simulink library "xrbsImage_r3"  (Simulink 5.1)
libraries: xbsIndex_r3 x24, xrbsDSP_r3 x5, xrbsImage_r3 x4
settings Model: Creator=singhj  LastModifiedBy=shirazi  ProdHWDeviceType=Microprocessor

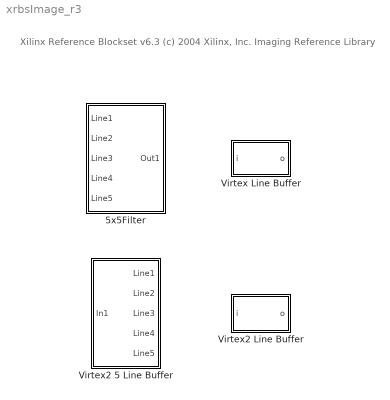
== system xrbsImage_r3 ==
  note: Xilinx Reference Blockset v6.3
      | (c) 2004  Xilinx, Inc.
      |
      | Imaging Reference Library
  5x5Filter : Subsystem  mask(5x5 Filter){maskNum=Edge, coef_n_bits=6, coef_bin_pt=0, smpl_n_bits=8, smpl_bin_pt=0, smpl_period=1, mask=0, maskDiv=0}
      mask prompts: maskNum "5x5 Mask"; coef_n_bits "Number of Bits per Coefficient"; coef_bin_pt "Binary Point for Coefficient"; smpl_n_bits "Number of Bits per Input Sample"; smpl_bin_pt "Binary Point for Input Samples"; smpl_period "Sample Period"; mask "Mask Value"; maskDiv "Mask Division"
      mask help: The Xilinx 5x5 Filter reference block is implemented using 5 n-tap MAC FIR Filters. Nine different 2-D filters have been provided to filter grayscale images.
      mask init:
      | [bg,fg] = xlcmap('XBlock',0);
      | iPos = get_param(gcb,'Position');
      | iWidth=iPos(3)-iPos(1); iHeight=iPos(4)-iPos(2);
      | iCx=iWidth/2;
      | iCy=iHeight/2;
      | [logoX, logoY] = xlogo(iPos);
      | 
      | % Different 5x5 Filters 
      | %  by default edge is used
      | 
      | edge = [ 0  0  0  0 0; ...
      |          0 -1 -1 -1 0; ...
      |          0 -1  8 -1 0; ...
      |          0 -1 -1 -1 0; ...
      |          0  0  0  0 0];
      | edgeDiv = 1;
      | 
      | sobelX = [ 0  0  0  0 0; ...
      |            0 -1  0  1 0; ...
      |            0 -2  0  2 0; ...
      |            0 -1  0  1 0; ...
      |            0  0  0  0 0];
      | sobelXDiv = 1;
      | 
      | sobelY = [ 0  0  0  0 0; ...
      |            0  1  2  1 0; ...
      |            0  0  0  0 0; ...
      |            0 -1 -2 -1 0; ...
      |            0  0  0  0 0];
      | sobelYDiv = 1;
      | 
      | sobelXY = [ 0  0  0  0 0; ...
      |             0  0 -1 -1 0; ...
      |             0  1  0 -1 0; ...
      |             0  1  1  0 0; ...
      |             0  0  0  0 0];
      | sobelXYDiv = 1;
      | 
      | blur = [ 1  1  1  1 1; ...
      |          1  0  0  0 1; ...
      |          1  0  0  0 1; ...
      |          1  0  0  0 1; ...
      |          1  1  1  1 1];
      | blurDiv = 1/16;
      | 
      | smooth = [ 1  1  1  1 1; ...
      |            1  5  5  5 1; ...
      |            1  5 44  5 1; ...
      |            1  5  5  5 1; ...
      |            1  1  1  1 1];
      | smoothDiv = 1/100;
      | 
      | sharpen = [ 0  0  0  0 0; ...
      |             0 -2 -2 -2 0; ...
      |             0 -2 32 -2 0; ...
      |             0 -2 -2 -2 0; ...
      |             0  0  0  0 0];
      | sharpenDiv = 1/16;
      | 
      | 
      | gaussian = [1 1 2 1 1; ...
      |             1 2 4 2 1; ...
      |             2 4 8 4 2; ...
      |             1 2 4 2 1; ...
      |             1 1 2 1 1];
      | gaussianDiv = 1/52;
      | 
      | identity = [ 0  0  0  0 0; ...
      |              0  0  0  0 0; ...
      |              0  0  1  0 0; ...
      |              0  0  0  0 0; ...
      |              0  0  0  0 0];
      | identityDiv = 1;
      | 
      | mask = zeros(5,5,5);
      | mask(:,:,1) = edge;
      | mask(:,:,2) = sobelX;
      | mask(:,:,3) = sobelY;
      | mask(:,:,4) = sobelXY;
      | mask(:,:,5) = blur;
      | mask(:,:,6) = smooth;
      | mask(:,:,7) = sharpen;
      | mask(:,:,8) = gaussian;
      | mask(:,:,9) = identity;
      | 
      | maskDiv = [edgeDiv sobelXDiv sobelYDiv sobelXYDiv blurDiv smoothDiv sharpenDiv gaussianDiv identityDiv];
      mask Help: eval('xlWeb(xlhtmldoclink(''5x5Filter''))');
      mask StyleString: popup(Edge|Sobel X|Sobel Y|Sobel X-Y|Blur|Smooth|Sharpen|Gaussian|Identity),edit,edit,edit,edit,edit,edit,edit
      mask Display:
      | patch([0 iWidth iWidth 0],[0 0 iHeight iHeight] , bg);
      | patch(logoX,logoY , fg);
      | port_label('input',1,'Line1');
      | port_label('input',2,'Line2');
      | port_label('input',3,'Line3');
      | port_label('input',4,'Line4');
      | port_label('input',5,'Line5');
      | port_label('output',1,'out');
      | plot([0 0 iWidth iWidth 0], [0 iHeight iHeight 0 0]);
  Virtex Line Buffer : Subsystem  mask(Virtex Line Buffer){buf_depth=64, cst=1}
      mask prompts: buf_depth "Buffer Depth"; cst "Sample Period"
      mask help: The Xilinx Virtex Line Buffer reference block delayes a sequential stream of pixels by the specified buffer depth.
      mask init:
      | str = sprintf('-%d',buf_depth);
      | [bg,fg] = xlcmap('XBlock',0);
      | iPos = get_param(gcb,'Position');
      | iWidth=iPos(3)-iPos(1); iHeight=iPos(4)-iPos(2);
      | iCx=iWidth/2;
      | iCy=iHeight/2;
      | [logoX, logoY] = xlogo(iPos);
      mask Help: eval('xlWeb(xlhtmldoclink(''Virtex Line Buffer''))');
      mask Display:
      | patch([0 iWidth iWidth 0],[0 0 iHeight iHeight] , bg);
      | patch(logoX,logoY , fg);
      | text(iCx-6,iCy,'z');
      | text(iCx,iCy+4,str);
      | plot([0 0 iWidth iWidth 0], [0 iHeight iHeight 0 0]);
  Virtex2 5 Line Buffer : Subsystem  mask(Virtex2 5 Line Buffer){line_size=64, cst=1}
      mask prompts: line_size "Line Size"; cst "Sample Period"
      mask help: The block buffers a sequential stream of pixels to construct 5 lines of output. Each line is delayed by N samples, where N is the length of the line. Line 1 is delayed 4*N samples, each of the following lines are delay by N fewer samples, and line 5 is a copy of the input.
      mask init:
      | [bg,fg] = xlcmap('XBlock',0);
      | iPos = get_param(gcb,'Position');
      | iWidth=iPos(3)-iPos(1); iHeight=iPos(4)-iPos(2);
      | iCx=iWidth/2;
      | iCy=iHeight/2;
      | [logoX, logoY] = xlogo(iPos);
      mask Help: eval('xlWeb(xlhtmldoclink(''Virtex2 5 Line Buffer''))');
      mask Display:
      | patch([0 iWidth iWidth 0],[0 0 iHeight iHeight] , bg);
      | patch(logoX,logoY , fg);
      | port_label('input',1,'in');
      | port_label('output',1,'Line1');
      | port_label('output',2,'Line2');
      | port_label('output',3,'Line3');
      | port_label('output',4,'Line4');
      | port_label('output',5,'Line5');
      | plot([0 0 iWidth iWidth 0], [0 iHeight iHeight 0 0]);
  Virtex2 Line Buffer : Subsystem  mask(Virtex2 Line Buffer){buf_depth=64, cst=1}
      mask prompts: buf_depth "Buffer Depth"; cst "Sample Period"
      mask help: The Xilinx Virtex2 Line Buffer reference block delayes a sequential stream of pixels by the specified buffer depth. It is optimized for the Virtex2 family since it uses the Read Before Write option on the underlying Single Port RAM block.
      mask init: same as xrbsImage_r3/Virtex Line Buffer
      mask Help: eval('xlWeb(xlhtmldoclink(''Virtex2 Line Buffer''))');
      mask Display:
      | patch([0 iWidth iWidth 0],[0 0 iHeight iHeight] , bg);
      | patch(logoX,logoY , fg);
      | text(iCx-6,iCy,'z');
      | text(iCx,iCy+4,str);
      | plot([0 0 iWidth iWidth 0], [0 iHeight iHeight 0 0]);

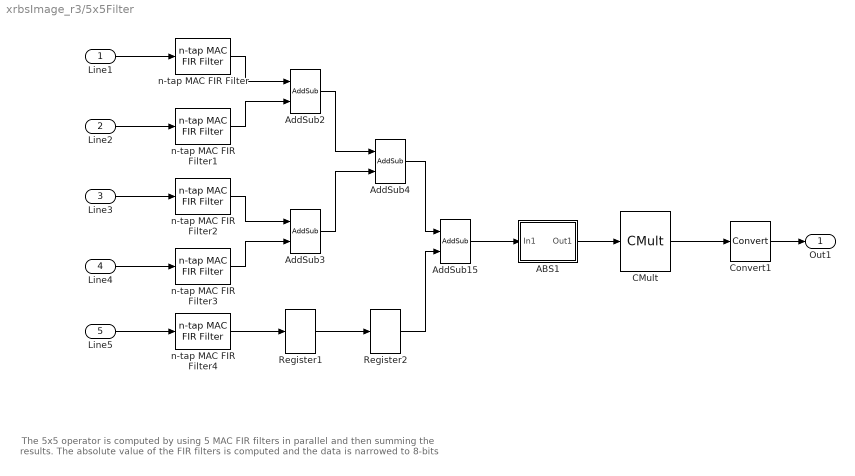
== system xrbsImage_r3/5x5Filter ==
  note: The 5x5 operator is computed by using 5 MAC FIR filters in parallel and then
      | summing the results.  The absolute value of the FIR filters is computed
      | and the data is narrowed to 8-bits
  Line1 : Inport
  Line2 : Inport  Port=2
  Line3 : Inport  Port=3
  Line4 : Inport  Port=4
  Line5 : Inport  Port=5
  ABS1 : Subsystem
  AddSub{2..4,15} (4 alike) : xbsIndex_r3/AddSub  mode=Addition  precision=Full  arith_type=Unsigned  n_bits=8  bin_pt=2  quantization=Truncate  overflow=Wrap  latency=1  explicit_period=off  period=1  en=off  dbl_ovrd=off  use_core=off  pipeline=off  use_rpm=off  gen_core=on
      settings: xl_area=[0, 0, 0, 0, 0, 0, 0]
  CMult : xbsIndex_r3/CMult  const=maskDiv(maskNum)  const_n_bits=18  const_bin_pt=17  precision=Full  arith_type=Unsigned  n_bits=8  bin_pt=0  quantization=Truncate  overflow=Wrap  mult_type=Parallel  mem_type=Distributed RAM  pipeline=on  latency=4  explicit_period=off  period=1  en=off  dbl_ovrd=off  oversample=2  use_rpm=off  placement_style=Rectangular Shape  gen_core=on
      settings: xl_area=[0, 0, 0, 0, 0, 0, 0]
  Convert1 : xbsIndex_r3/Convert  arith_type=Unsigned  n_bits=8  bin_pt=0  quantization=Truncate  overflow=Saturate  latency=1  explicit_period=off  period=1  dbl_ovrd=off  inserted_by_tool=off
      settings: xl_area=[0, 0, 0, 0, 0, 0, 0]
  Register1 : xbsIndex_r3/Register  init=0  reg_only_valid=off  explicit_period=off  period=1  rst=off  en=off  out_en=off  dbl_ovrd=off
      settings: xl_area=[0, 0, 0, 0, 0, 0, 0]
  Register2 : xbsIndex_r3/Register  init=0  reg_only_valid=off  explicit_period=off  period=1  rst=off  en=off  out_en=off  dbl_ovrd=off
      settings: xl_area=[0, 0, 0, 0, 0, 0, 0]
  n-tap MAC FIR Filter : xrbsDSP_r3/n-tap MAC FIR Filter  coef=mask(1,5:-1:1,maskNum)  coef_n_bits=coef_n_bits  coef_bin_pt=coef_bin_pt  smpl_n_bits=smpl_n_bits  smpl_bin_pt=smpl_bin_pt  smpl_period=smpl_period
  n-tap MAC FIR Filter1 : xrbsDSP_r3/n-tap MAC FIR Filter  coef=mask(2,5:-1:1,maskNum)  coef_n_bits=coef_n_bits  coef_bin_pt=coef_bin_pt  smpl_n_bits=smpl_n_bits  smpl_bin_pt=smpl_bin_pt  smpl_period=smpl_period
  n-tap MAC FIR Filter2 : xrbsDSP_r3/n-tap MAC FIR Filter  coef=mask(3,5:-1:1,maskNum)  coef_n_bits=coef_n_bits  coef_bin_pt=coef_bin_pt  smpl_n_bits=smpl_n_bits  smpl_bin_pt=smpl_bin_pt  smpl_period=smpl_period
  n-tap MAC FIR Filter3 : xrbsDSP_r3/n-tap MAC FIR Filter  coef=mask(4,5:-1:1,maskNum)  coef_n_bits=coef_n_bits  coef_bin_pt=coef_bin_pt  smpl_n_bits=smpl_n_bits  smpl_bin_pt=smpl_bin_pt  smpl_period=smpl_period
  n-tap MAC FIR Filter4 : xrbsDSP_r3/n-tap MAC FIR Filter  coef=mask(5,5:-1:1,maskNum)  coef_n_bits=coef_n_bits  coef_bin_pt=coef_bin_pt  smpl_n_bits=smpl_n_bits  smpl_bin_pt=smpl_bin_pt  smpl_period=smpl_period
  Out1 : Outport
  wires:
  Line1/1 -> n-tap MAC FIR Filter/1
  Line2/1 -> n-tap MAC FIR Filter1/1
  Line3/1 -> n-tap MAC FIR Filter2/1
  Line4/1 -> n-tap MAC FIR Filter3/1
  Line5/1 -> n-tap MAC FIR Filter4/1
  n-tap MAC FIR Filter/1 -> AddSub2/1
  n-tap MAC FIR Filter1/1 -> AddSub2/2
  n-tap MAC FIR Filter2/1 -> AddSub3/1
  n-tap MAC FIR Filter3/1 -> AddSub3/2
  AddSub2/1 -> AddSub4/1
  AddSub3/1 -> AddSub4/2
  n-tap MAC FIR Filter4/1 -> Register1/1
  Register1/1 -> Register2/1
  AddSub15/1 -> ABS1/1(In1)
  AddSub4/1 -> AddSub15/1
  Register2/1 -> AddSub15/2
  CMult/1 -> Convert1/1
  ABS1/1(Out1) -> CMult/1
  Convert1/1 -> Out1/1

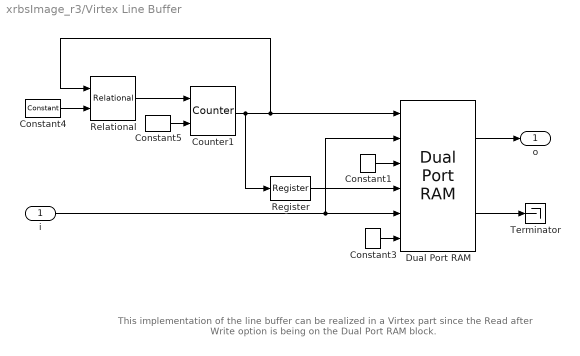
== system xrbsImage_r3/Virtex Line Buffer ==
  note: This implementation of the line buffer can be realized in a Virtex
      | part since the Read after Write option is being on the
      |  Dual Port RAM block.
  i : Inport
  Constant1 : xbsIndex_r3/Constant  const=0  arith_type=Boolean  n_bits=1  bin_pt=0  explicit_period=off  period=cst  dbl_ovrd=off
  Constant3 : xbsIndex_r3/Constant  const=1  arith_type=Boolean  n_bits=1  bin_pt=0  explicit_period=off  period=cst  dbl_ovrd=off
  Constant4 : xbsIndex_r3/Constant  const=buf_depth-1  arith_type=Unsigned  n_bits=ceil(log2(buf_depth))  bin_pt=0  explicit_period=off  period=cst  dbl_ovrd=off
  Constant5 : xbsIndex_r3/Constant  const=0  arith_type=Unsigned  n_bits=ceil(log2(buf_depth))  bin_pt=0  explicit_period=on  period=cst  dbl_ovrd=off
  Counter1 : xbsIndex_r3/Counter  cnt_type=Free Running  n_bits=ceil(log2(buf_depth))  bin_pt=0  arith_type=Unsigned  start_count=1  cnt_to=buf_depth -1  cnt_by_val=1  operation=Up  explicit_period=off  period=cst  load_pin=on  rst=off  en=off  dbl_ovrd=off  gen_core=on  use_rpm=off
      settings: xl_area=[6 10 0 11 0 0 0]
  Dual Port RAM : xbsIndex_r3/Dual Port RAM  depth=buf_depth  initVector=0  write_mode_A=Read After Write  write_mode_B=Read After Write  latency=1  mem_collision=off  init_zero=on  explicit_period=off  period=-1  dbl_ovrd=off  gen_core=on
      settings: xl_area=[0 0 1 0 0 0 0]
  Register : xbsIndex_r3/Register  init=0  reg_only_valid=off  explicit_period=off  period=1  rst=off  en=off  out_en=off  dbl_ovrd=off
      settings: xl_area=[5 10 0 0 0 0 0]
  Relational : xbsIndex_r3/Relational  mode=a=b  latency=0  explicit_period=on  period=cst  en=off  dbl_ovrd=off
      settings: xl_area=[4 0 0 3 0 0 0]
  Terminator : Terminator
  o : Outport
  wires:
  Dual Port RAM/2 -> Terminator/1
  i/1 -> Dual Port RAM/5, Dual Port RAM/2
  Dual Port RAM/1 -> o/1
  Constant3/1 -> Dual Port RAM/6
  Constant1/1 -> Dual Port RAM/3
  Counter1/1 -> Relational/1, Dual Port RAM/1, Register/1
  Relational/1 -> Counter1/1
  Constant4/1 -> Relational/2
  Register/1 -> Dual Port RAM/4
  Constant5/1 -> Counter1/2

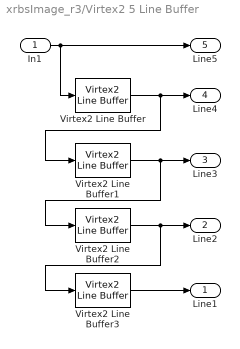
== system xrbsImage_r3/Virtex2 5 Line Buffer ==
  In1 : Inport
  Virtex2 Line Buffer{,1..3} (4 alike) : xrbsImage_r3/Virtex2 Line Buffer  buf_depth=line_size  cst=cst
  Line1 : Outport
  Line2 : Outport  Port=2
  Line3 : Outport  Port=3
  Line4 : Outport  Port=4
  Line5 : Outport  Port=5
  wires:
  In1/1 -> Line5/1, Virtex2 Line Buffer/1
  Virtex2 Line Buffer/1 -> Line4/1, Virtex2 Line Buffer1/1
  Virtex2 Line Buffer1/1 -> Line3/1, Virtex2 Line Buffer2/1
  Virtex2 Line Buffer2/1 -> Line2/1, Virtex2 Line Buffer3/1
  Virtex2 Line Buffer3/1 -> Line1/1

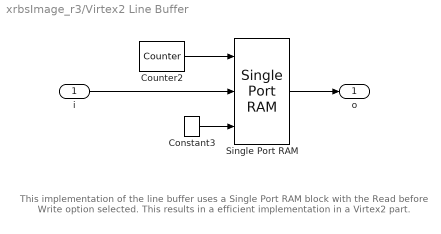
== system xrbsImage_r3/Virtex2 Line Buffer ==
  note: This implementation of the line buffer uses a
      |  Single Port RAM block with the Read before Write
      | option selected.  This results in a efficient
      | implementation in a Virtex2 part.
  i : Inport
  Constant3 : xbsIndex_r3/Constant  const=1  arith_type=Boolean  n_bits=1  bin_pt=0  explicit_period=on  period=cst  dbl_ovrd=off
  Counter2 : xbsIndex_r3/Counter  cnt_type=Count Limited  n_bits=ceil(log2(buf_depth-1))  bin_pt=0  arith_type=Unsigned  start_count=0  cnt_to=buf_depth -2  cnt_by_val=1  operation=Up  explicit_period=on  period=cst  load_pin=off  rst=off  en=off  dbl_ovrd=off  gen_core=on  use_rpm=off
      settings: xl_area=[7 10 0 13 0 0 0]
  Single Port RAM : xbsIndex_r3/Single Port RAM  depth=buf_depth-1  initVector=0  write_mode=Read Before Write  latency=1  distributed_mem=off  init_zero=on  explicit_period=off  period=1  en=off  dbl_ovrd=off  gen_core=on  use_rpm=off
      settings: xl_area=[0 0 1 0 0 0 0]
  o : Outport
  wires:
  Constant3/1 -> Single Port RAM/3
  Single Port RAM/1 -> o/1
  i/1 -> Single Port RAM/2
  Counter2/1 -> Single Port RAM/1

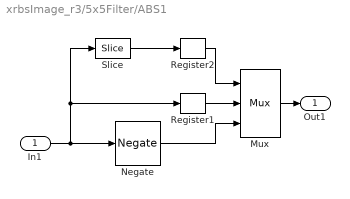
== system xrbsImage_r3/5x5Filter/ABS1 ==
  In1 : Inport
  Mux : xbsIndex_r3/Mux  inputs=2  precision=Full  arith_type=Unsigned  n_bits=8  bin_pt=0  quantization=Truncate  overflow=Saturate  latency=1  mux_type=off  explicit_period=off  period=1  en=off  dbl_ovrd=off  gen_core=on  use_rpm=off
      settings: xl_area=[0, 0, 0, 0, 0, 0, 0]
  Negate : xbsIndex_r3/Negate  precision=Full  arith_type=Unsigned  n_bits=8  bin_pt=2  quantization=Truncate  overflow=Wrap  latency=1  explicit_period=off  period=1  en=off  dbl_ovrd=off  use_core=off  gen_core=on  use_rpm=off
      settings: xl_area=[0, 0, 0, 0, 0, 0, 0]
  Register1 : xbsIndex_r3/Register  init=0  reg_only_valid=off  explicit_period=off  period=1  rst=off  en=off  out_en=off  dbl_ovrd=off
      settings: xl_area=[0, 0, 0, 0, 0, 0, 0]
  Register2 : xbsIndex_r3/Register  init=0  reg_only_valid=off  explicit_period=off  period=1  rst=off  en=off  out_en=off  dbl_ovrd=off
      settings: xl_area=[0, 0, 0, 0, 0, 0, 0]
  Slice : xbsIndex_r3/Slice  mode=Upper Bit Location + Width  nbits=1  bit1=0  base1=MSB of Input  bit0=0  base0=LSB of Input  boolean_output=off  explicit_period=off  period=1  dbl_ovrd=off
  Out1 : Outport
  wires:
  Register1/1 -> Mux/2
  Register2/1 -> Mux/1
  Mux/1 -> Out1/1
  In1/1 -> Register1/1, Slice/1, Negate/1
  Negate/1 -> Mux/3
  Slice/1 -> Register2/1
